simulink library "libbha_io"  (R2015b)
settings: Solver=FixedStepDiscrete  StartTime=0.0  StopTime=Inf  FixedStep=0.004  RelTol=1e-3
PostLoadFcn:
  | , if any(exist('dsrtsu_mdlpostloadfcn', 'file') == [2, 3, 6]), try dsrtsu_mdlpostloadfcn('Execute', bdroot); catch fprintf('Error in PostLoadFcn (dsrtsu_mdlpostloadfcn) for model "%s":\n %s\n', bdroot, lasterr); end, end,
libraries: libbha_io x33, libc_filters_diff x8, libc_bitoperations x8, simulink x7
settings Model: DSRTSU_INTERNAL_RTI_VER=470  DSRTSU_INTERNAL_RTI_TYPE=rti1007  DSRTSU_INTERNAL_RTIFPGA=60  Creator=Falkenhahn  LastModifiedBy=fav
settings DataIOCC: SaveFormat=Array
settings OptimizationCC: BlockReduction=off  OptimizeBlockIOStorage=off  BufferReuse=off  GlobalBufferReuse=off  ExpressionFolding=off  LocalBlockOutputs=off
settings DebuggingCC: UnderspecifiedInitializationDetection=Classic  MergeDetectMultiDrivingBlocksExec=none  SolverPrmCheckMsg=warning
settings HardwareCC: ProdBitPerPointer=32  ProdLargestAtomicFloat=None  ProdEndianess=BigEndian  ProdWordSize=32  ProdHWDeviceType=Generic->Custom  TargetIntDivRoundTo=Zero  TargetEndianess=BigEndian  TargetHWDeviceType=Generic->Custom
settings RTWCC: SystemTargetFile=rti1007.tlc  MakeCommand=make_rti  TemplateMakefile=rti1007.tmf  Description=dSPACE DS1007 Hardware Platform
settings STFCustomTargetCC: ParMdlRefBuildCompliant=on  ConcurrentExecutionCompliant=off  MatFileLogging=on  SystemTargetFile=rti1007.tlc
settings GRTTargetCC: CompOptLevelCompliant=off  ConcurrentExecutionCompliant=off  GeneratePreprocessorConditionals=Disable all  CombineOutputUpdateFcns=off  GRTInterface=on  UseToolchainInfoCompliant=off  ExtModeMexFile=noextcomm
settings ConfigComp: CovModelRefEnable=Off

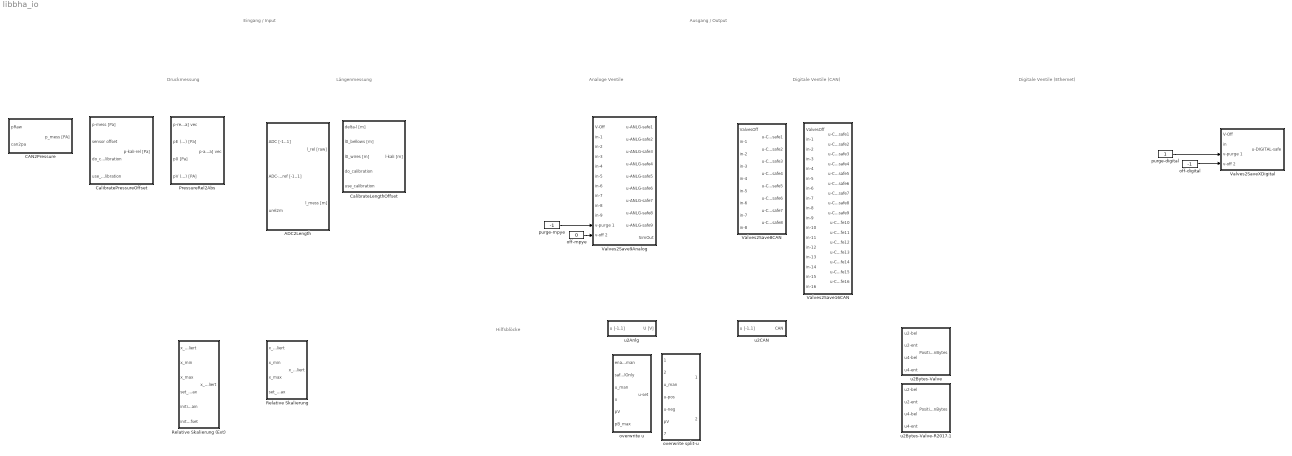
== system libbha_io ==
  note: Druckmessung
  note: Längenmessung
  note: Analoge Ventile
  note: Digitale Ventile (CAN)
  note: Hilfsblöcke
  note: Eingang / Input
  note: Ausgang / Output
  note: Digitale Ventile (Ethernet)
  ADC2Length : Subsystem
  CAN2Pressure : Subsystem
  CalibrateLengthOffset : Subsystem
  CalibratePressureOffset : Subsystem
  PressureRel2Abs : Subsystem
  Relative Skalierung : Subsystem  mask{x_min_init=1e5, x_max_init=2e5}
      mask prompts: x_min_init "x min init"; x_max_init "x max init"
      settings: AttributesFormatString=|
      | Quick-and-dirty Kalibrierung:
      | Passt unskalierte Messgrößen
      | in Zuständen entlüftet (-1) und belüftet (1)
      | auf Minimal- bzw. Maximalwert an
      | 
      | Initialisierung verbesserungswürdig
  Relative Skalierung (Ext) : Subsystem  mask{x_min_init=1e5, x_max_init=2e5}
      mask prompts: x_min_init "x min init"; x_max_init "x max init"
      settings: AttributesFormatString=|
      | Quick-and-dirty Kalibrierung:
      | Passt unskalierte Messgrößen
      | in Zuständen entlüftet (-1) und belüftet (1)
      | auf Minimal- bzw. Maximalwert an
  Valves2Save16CAN : Subsystem
  Valves2Save8CAN : Subsystem
  Valves2Save9Analog : Subsystem
  Valves2SaveXDigital : Subsystem
  off-digital : Constant  Value=-1
  off-mpye : Constant  Value=0
      settings: AttributesFormatString=|
      | mpye: 0
      | mhe: -1 (ambient)
  overwrite split-u : Subsystem
  overwrite u : Subsystem
  purge-digital : Constant
  purge-mpye : Constant  Value=-1
      settings: AttributesFormatString=|
      | mpye -1
      | mhe: 1
  u2Anlg : Subsystem
  u2Bytes-Valve : Subsystem
  u2Bytes-Valve-R2017.1 : Subsystem
  u2CAN : Subsystem
  wires:
  purge-mpye/1 -> Valves2Save9Analog/11(v-purge 1)
  off-mpye/1 -> Valves2Save9Analog/12(v-off 2)
  purge-digital/1 -> Valves2SaveXDigital/3(v-purge 1)
  off-digital/1 -> Valves2SaveXDigital/4(v-off 2)

== system libbha_io/ADC2Length ==
  ADC [-1..1] : Inport
  ADC-U-ref [-1..1] : Inport  Port=2
  urel2m : Inport  Port=3
  Divide : Product  Inputs=*/
  Product : Product  RndMeth=Zero
  Saturation > 0 : Saturate  UpperLimit=inf  LowerLimit=0.001
  l_rel [raw] : Outport
  l_mess [m] : Outport  Port=2
  wires:
  urel2m/1 -> Product/2
  Divide/1 -> Product/1, l_rel [raw]/1
  Product/1 -> l_mess [m]/1
  Saturation > 0/1 -> Divide/2
  ADC [-1..1]/1 -> Divide/1
  ADC-U-ref [-1..1]/1 -> Saturation > 0/1

== system libbha_io/CAN2Pressure ==
  pRaw : Inport
  can2pa : Inport  Port=2
  Data Type Conversion : DataTypeConversion  OutDataTypeStr=double  RndMeth=Nearest
  Product : Product  RndMeth=Zero
  p_mess [PA] : Outport
  wires:
  Product/1 -> p_mess [PA]/1
  can2pa/1 -> Product/2
  Data Type Conversion/1 -> Product/1
  pRaw/1 -> Data Type Conversion/1

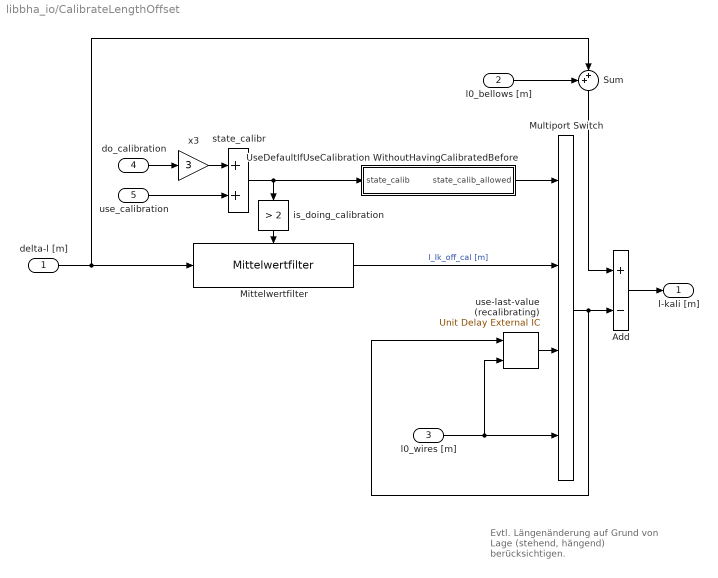
== system libbha_io/CalibrateLengthOffset ==
  note: Evtl. Längenänderung auf Grund von
      | Lage (stehend, hängend) berücksichtigen.
  delta-l [m] : Inport
  l0_bellows [m] : Inport  Port=2
  l0_wires [m] : Inport  Port=3
  do_calibration : Inport  Port=4
  use_calibration : Inport  Port=5
  Add : Sum  Inputs=+-
  Mittelwertfilter : libc_filters_diff/Mittelwertfilter
      settings: AttributesFormatString=Eingangs-Mittelwertbildung wenn aktiviert,\nandernfalls wird Mittelwert gehalten & ausgegeben
  Multiport Switch : MultiPortSwitch  Inputs=2  DataPortForDefault=Additional data port  DiagnosticForDefault=None
  Sum : Sum  Inputs=++|
  UseDefaultIfUseCalibration WithoutHavingCalibratedBefore : Subsystem
  is_doing_calibration : simulink/Logic and Bit Operations/Compare To Constant  relop=>  const=2  OutDataTypeStr=uint8
  state_calibr : Sum
      settings: AttributesFormatString=|
      | 0 = use default
      | 1 = use calibration
      | 2 > do calibration
  use-last-value (recalibrating) : simulink/Additional Math & Discrete/Additional Discrete/Unit Delay External IC  tsamp=-1
  x3 : Gain  Gain=3
  "l-kali [m] " : Outport
  wires:
  use-last-value (recalibrating)/1 -> Multiport Switch/3
  is_doing_calibration/1 -> Mittelwertfilter/Enable
  l0_wires [m]/1 -> use-last-value (recalibrating)/2, Multiport Switch/4
  Multiport Switch/1 -> use-last-value (recalibrating)/1, Add/2
  state_calibr/1 -> UseDefaultIfUseCalibration WithoutHavingCalibratedBefore/1(state_calib), is_doing_calibration/1
  delta-l [m]/1 -> Mittelwertfilter/1, Sum/2
  do_calibration/1 -> x3/1
  x3/1 -> state_calibr/1
  use_calibration/1 -> state_calibr/2
  Add/1 -> "l-kali [m] "/1
  Mittelwertfilter/1 -> Multiport Switch/2  "l_Ik_off_cal [m]"
  Sum/1 -> Add/1
  l0_bellows [m]/1 -> Sum/1
  UseDefaultIfUseCalibration WithoutHavingCalibratedBefore/1(state_calib_allowed) -> Multiport Switch/1

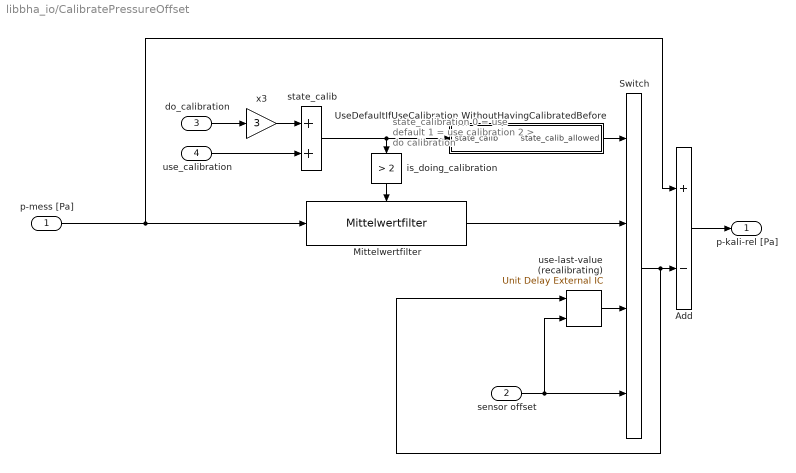
== system libbha_io/CalibratePressureOffset ==
  note: state_calibration
      | 0 = use default
      | 1 = use calibration
      | 2 > do calibration
  p-mess [Pa] : Inport
  sensor offset : Inport  Port=2
  do_calibration : Inport  Port=3
  use_calibration : Inport  Port=4
  Add : Sum  Inputs=+-
  Mittelwertfilter : libc_filters_diff/Mittelwertfilter
      settings: AttributesFormatString=Eingangs-Mittelwertbildung wenn aktiviert,\nandernfalls wird Mittelwert gehalten & ausgegeben
  Switch : MultiPortSwitch  Inputs=2  DataPortForDefault=Additional data port  DiagnosticForDefault=None
  UseDefaultIfUseCalibration WithoutHavingCalibratedBefore : Subsystem
  is_doing_calibration : simulink/Logic and Bit Operations/Compare To Constant  relop=>  const=2  OutDataTypeStr=uint8
  state_calib : Sum
  use-last-value (recalibrating) : simulink/Additional Math & Discrete/Additional Discrete/Unit Delay External IC  tsamp=-1
  x3 : Gain  Gain=3
  p-kali-rel [Pa] : Outport
  wires:
  use_calibration/1 -> state_calib/2
  x3/1 -> state_calib/1
  state_calib/1 -> UseDefaultIfUseCalibration WithoutHavingCalibratedBefore/1(state_calib), is_doing_calibration/1
  Switch/1 -> use-last-value (recalibrating)/1, Add/2
  sensor offset/1 -> use-last-value (recalibrating)/2, Switch/4
  Mittelwertfilter/1 -> Switch/2
  is_doing_calibration/1 -> Mittelwertfilter/Enable
  use-last-value (recalibrating)/1 -> Switch/3
  UseDefaultIfUseCalibration WithoutHavingCalibratedBefore/1(state_calib_allowed) -> Switch/1
  Add/1 -> p-kali-rel [Pa]/1
  p-mess [Pa]/1 -> Mittelwertfilter/1, Add/1
  do_calibration/1 -> x3/1

== system libbha_io/PressureRel2Abs ==
  p-rel [Pa] vec : Inport
  pE (min) [Pa] : Inport  Port=2
  p0 [Pa] : Inport  Port=3
  pV (max) [PA] : Inport  Port=4
  Saturation Dynamic : simulink/Discontinuities/Saturation Dynamic  OutMin=[]  OutMax=[]  OutDataTypeStr=Inherit: Same as second input  OutDataType=fixdt(1, 16)  OutScaling=2^-10  DoSatur=off
  Sum : Sum  Inputs=|++
  do not allow pressures close to zero : Saturate  UpperLimit=inf  LowerLimit=0.11e5
  p-abs [Pa] vec : Outport
  wires:
  do not allow pressures close to zero/1 -> p-abs [Pa] vec/1
  Saturation Dynamic/1 -> do not allow pressures close to zero/1
  p0 [Pa]/1 -> Sum/2
  Sum/1 -> Saturation Dynamic/2
  pV (max) [PA]/1 -> Saturation Dynamic/1
  p-rel [Pa] vec/1 -> Sum/1  "l_meas_11"
  pE (min) [Pa]/1 -> Saturation Dynamic/3

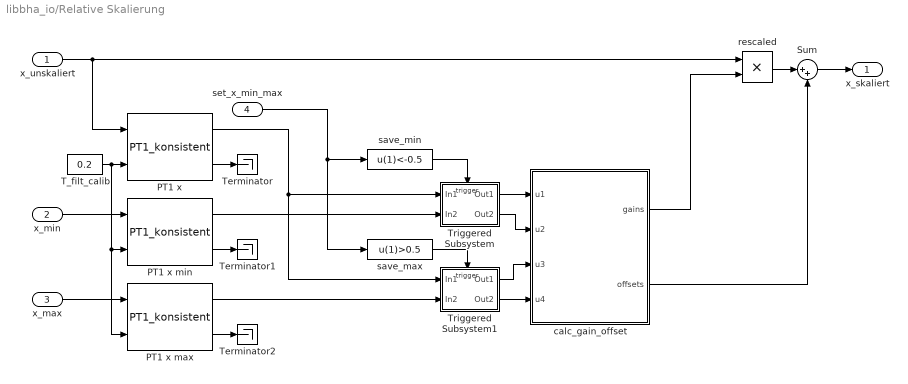
== system libbha_io/Relative Skalierung ==
  x_unskaliert : Inport
  x_min : Inport  Port=2
  x_max : Inport  Port=3
  set_x_min_max : Inport  Port=4
  PT1 x : libc_filters_diff/PT1_konsistent
  PT1 x max : libc_filters_diff/PT1_konsistent
  PT1 x min : libc_filters_diff/PT1_konsistent
  Sum : Sum  Inputs=|++
  T_filt_calib : Constant  Value=0.2
  Terminator : Terminator
  Terminator1 : Terminator
  Terminator2 : Terminator
  Triggered Subsystem : Subsystem  TreatAsAtomicUnit=on
  Triggered Subsystem1 : Subsystem  TreatAsAtomicUnit=on
  calc_gain_offset : MATLAB Function  TreatAsAtomicUnit=on
  rescaled : Product  Inputs=**  RndMeth=Zero
  save_max : Fcn  Expr=u(1)>0.5
  save_min : Fcn  Expr=u(1)<-0.5
  x_skaliert : Outport
  wires:
  PT1 x/1 -> Triggered Subsystem/1(In1), Triggered Subsystem1/1(In1)
  x_min/1 -> PT1 x min/1
  save_max/1 -> Triggered Subsystem1/Trigger
  x_unskaliert/1 -> PT1 x/1, rescaled/1
  set_x_min_max/1 -> save_max/1, save_min/1
  rescaled/1 -> Sum/1
  Sum/1 -> x_skaliert/1
  calc_gain_offset/1(gains) -> rescaled/2
  calc_gain_offset/2(offsets) -> Sum/2
  PT1 x min/1 -> Triggered Subsystem/2(In2)
  PT1 x max/1 -> Triggered Subsystem1/2(In2)
  save_min/1 -> Triggered Subsystem/Trigger
  x_max/1 -> PT1 x max/1
  T_filt_calib/1 -> PT1 x min/2, PT1 x max/2, PT1 x/2
  PT1 x/2 -> Terminator/1
  PT1 x min/2 -> Terminator1/1
  PT1 x max/2 -> Terminator2/1
  Triggered Subsystem/1(Out1) -> calc_gain_offset/1(u1)
  Triggered Subsystem/2(Out2) -> calc_gain_offset/2(u2)
  Triggered Subsystem1/2(Out2) -> calc_gain_offset/4(u4)
  Triggered Subsystem1/1(Out1) -> calc_gain_offset/3(u3)

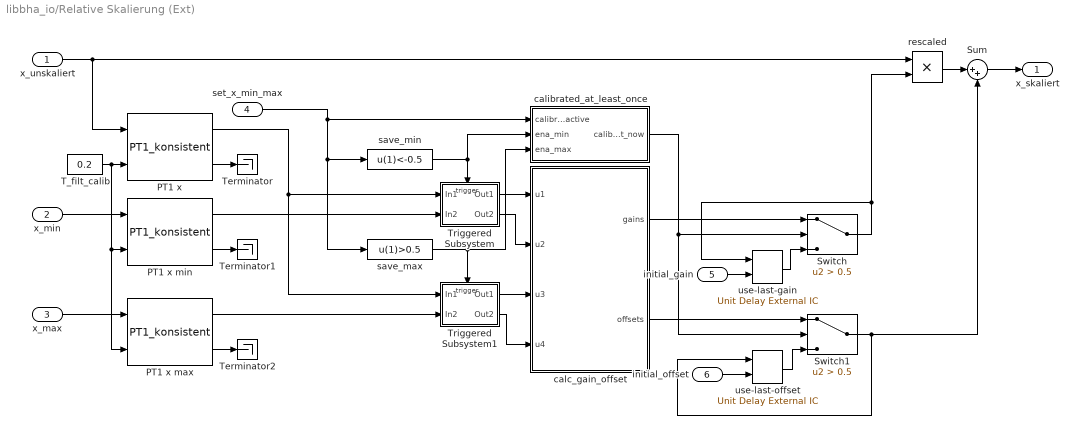
== system libbha_io/Relative Skalierung (Ext) ==
  x_unskaliert : Inport
  x_min : Inport  Port=2
  x_max : Inport  Port=3
  set_x_min_max : Inport  Port=4
  initial_gain : Inport  Port=5
  initial_offset : Inport  Port=6
  PT1 x : libc_filters_diff/PT1_konsistent
  PT1 x max : libc_filters_diff/PT1_konsistent
  PT1 x min : libc_filters_diff/PT1_konsistent
  Sum : Sum  Inputs=|++
  Switch : Switch  Criteria=u2 > Threshold  Threshold=0.5
  Switch1 : Switch  Criteria=u2 > Threshold  Threshold=0.5
  T_filt_calib : Constant  Value=0.2
  Terminator : Terminator
  Terminator1 : Terminator
  Terminator2 : Terminator
  Triggered Subsystem : Subsystem  TreatAsAtomicUnit=on
  Triggered Subsystem1 : Subsystem  TreatAsAtomicUnit=on
  calc_gain_offset : MATLAB Function  TreatAsAtomicUnit=on
  calibrated_at_least_once : Subsystem
  rescaled : Product  Inputs=**  RndMeth=Zero
  save_max : Fcn  Expr=u(1)>0.5
  save_min : Fcn  Expr=u(1)<-0.5
  use-last-gain : simulink/Additional Math & Discrete/Additional Discrete/Unit Delay External IC  tsamp=-1
  use-last-offset : simulink/Additional Math & Discrete/Additional Discrete/Unit Delay External IC  tsamp=-1
  x_skaliert : Outport
  wires:
  Triggered Subsystem1/1(Out1) -> calc_gain_offset/3(u3)
  Triggered Subsystem1/2(Out2) -> calc_gain_offset/4(u4)
  Triggered Subsystem/2(Out2) -> calc_gain_offset/2(u2)
  Triggered Subsystem/1(Out1) -> calc_gain_offset/1(u1)
  PT1 x max/2 -> Terminator2/1
  PT1 x min/2 -> Terminator1/1
  PT1 x/2 -> Terminator/1
  T_filt_calib/1 -> PT1 x/2, PT1 x max/2, PT1 x min/2
  x_max/1 -> PT1 x max/1
  save_min/1 -> calibrated_at_least_once/2(ena_min), Triggered Subsystem/Trigger
  PT1 x max/1 -> Triggered Subsystem1/2(In2)
  PT1 x min/1 -> Triggered Subsystem/2(In2)
  Switch1/1 -> Sum/2, use-last-offset/1
  Switch/1 -> rescaled/2, use-last-gain/1
  Sum/1 -> x_skaliert/1
  rescaled/1 -> Sum/1
  set_x_min_max/1 -> save_min/1, save_max/1, calibrated_at_least_once/1(calibration_active)
  x_unskaliert/1 -> rescaled/1, PT1 x/1
  save_max/1 -> calibrated_at_least_once/3(ena_max), Triggered Subsystem1/Trigger
  x_min/1 -> PT1 x min/1
  PT1 x/1 -> Triggered Subsystem1/1(In1), Triggered Subsystem/1(In1)
  initial_gain/1 -> use-last-gain/2
  calc_gain_offset/1(gains) -> Switch/1
  calibrated_at_least_once/1(calib_once_not_now) -> Switch1/2, Switch/2
  use-last-gain/1 -> Switch/3
  calc_gain_offset/2(offsets) -> Switch1/1
  initial_offset/1 -> use-last-offset/2
  use-last-offset/1 -> Switch1/3

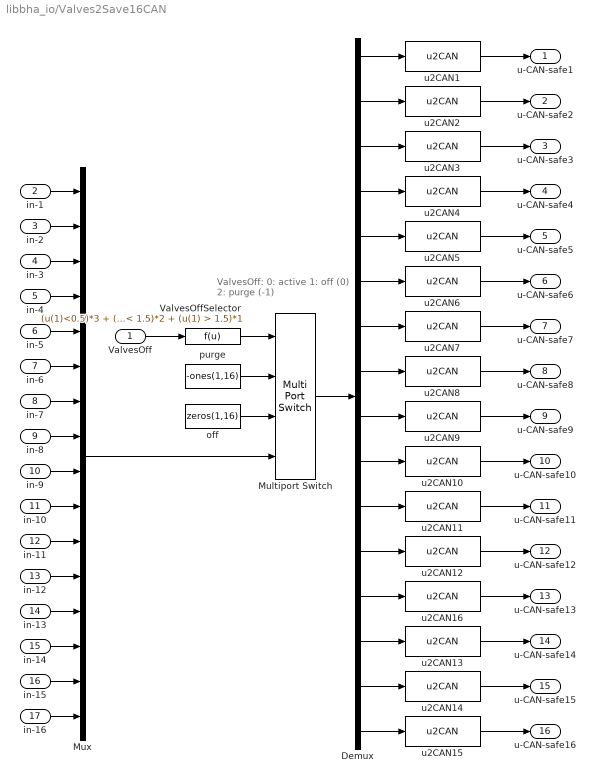
== system libbha_io/Valves2Save16CAN ==
  note: ValvesOff:
      | 0: active
      | 1: off (0)
      | 2: purge (-1)
  ValvesOff : Inport
  in-1 : Inport  Port=2
  in-2 : Inport  Port=3
  in-3 : Inport  Port=4
  in-4 : Inport  Port=5
  in-5 : Inport  Port=6
  in-6 : Inport  Port=7
  in-7 : Inport  Port=8
  in-8 : Inport  Port=9
  in-9 : Inport  Port=10
  in-10 : Inport  Port=11
  in-11 : Inport  Port=12
  in-12 : Inport  Port=13
  in-13 : Inport  Port=14
  in-14 : Inport  Port=15
  in-15 : Inport  Port=16
  in-16 : Inport  Port=17
  Demux : Demux  Outputs=16
  Multiport Switch : MultiPortSwitch
  Mux : Mux  Inputs=16
  ValvesOffSelector : Fcn  Expr=(u(1)<0.5)*3 + (u(1) >0.5)*(u(1) < 1.5)*2 + (u(1) > 1.5)*1
  off : Constant  Value=zeros(1,16)
  purge : Constant  Value=-ones(1,16)
  u2CAN{1..16} (16 alike) : libbha_io/u2CAN
  u-CAN-safe1 : Outport
  u-CAN-safe2 : Outport  Port=2
  u-CAN-safe3 : Outport  Port=3
  u-CAN-safe4 : Outport  Port=4
  u-CAN-safe5 : Outport  Port=5
  u-CAN-safe6 : Outport  Port=6
  u-CAN-safe7 : Outport  Port=7
  u-CAN-safe8 : Outport  Port=8
  u-CAN-safe9 : Outport  Port=9
  u-CAN-safe10 : Outport  Port=10
  u-CAN-safe11 : Outport  Port=11
  u-CAN-safe12 : Outport  Port=12
  u-CAN-safe13 : Outport  Port=13
  u-CAN-safe14 : Outport  Port=14
  u-CAN-safe15 : Outport  Port=15
  u-CAN-safe16 : Outport  Port=16
  wires:
  u2CAN8/1 -> u-CAN-safe8/1
  u2CAN7/1 -> u-CAN-safe7/1
  u2CAN6/1 -> u-CAN-safe6/1
  u2CAN5/1 -> u-CAN-safe5/1
  u2CAN4/1 -> u-CAN-safe4/1
  u2CAN3/1 -> u-CAN-safe3/1
  u2CAN2/1 -> u-CAN-safe2/1
  u2CAN1/1 -> u-CAN-safe1/1
  Demux/8 -> u2CAN8/1
  Demux/7 -> u2CAN7/1
  Demux/6 -> u2CAN6/1
  Demux/5 -> u2CAN5/1
  Demux/4 -> u2CAN4/1
  Demux/3 -> u2CAN3/1
  Demux/2 -> u2CAN2/1
  Demux/1 -> u2CAN1/1
  in-8/1 -> Mux/8
  in-7/1 -> Mux/7
  in-6/1 -> Mux/6
  in-5/1 -> Mux/5
  in-4/1 -> Mux/4
  in-3/1 -> Mux/3
  in-2/1 -> Mux/2
  in-1/1 -> Mux/1
  ValvesOff/1 -> ValvesOffSelector/1
  Mux/1 -> Multiport Switch/4
  Multiport Switch/1 -> Demux/1
  off/1 -> Multiport Switch/3
  purge/1 -> Multiport Switch/2
  ValvesOffSelector/1 -> Multiport Switch/1
  in-9/1 -> Mux/9
  in-10/1 -> Mux/10
  in-11/1 -> Mux/11
  in-12/1 -> Mux/12
  in-13/1 -> Mux/13
  in-14/1 -> Mux/14
  in-15/1 -> Mux/15
  in-16/1 -> Mux/16
  u2CAN9/1 -> u-CAN-safe9/1
  Demux/9 -> u2CAN9/1
  u2CAN10/1 -> u-CAN-safe10/1
  u2CAN11/1 -> u-CAN-safe11/1
  u2CAN12/1 -> u-CAN-safe12/1
  u2CAN16/1 -> u-CAN-safe13/1
  u2CAN13/1 -> u-CAN-safe14/1
  u2CAN14/1 -> u-CAN-safe15/1
  u2CAN15/1 -> u-CAN-safe16/1
  Demux/10 -> u2CAN10/1
  Demux/11 -> u2CAN11/1
  Demux/12 -> u2CAN12/1
  Demux/13 -> u2CAN16/1
  Demux/14 -> u2CAN13/1
  Demux/15 -> u2CAN14/1
  Demux/16 -> u2CAN15/1

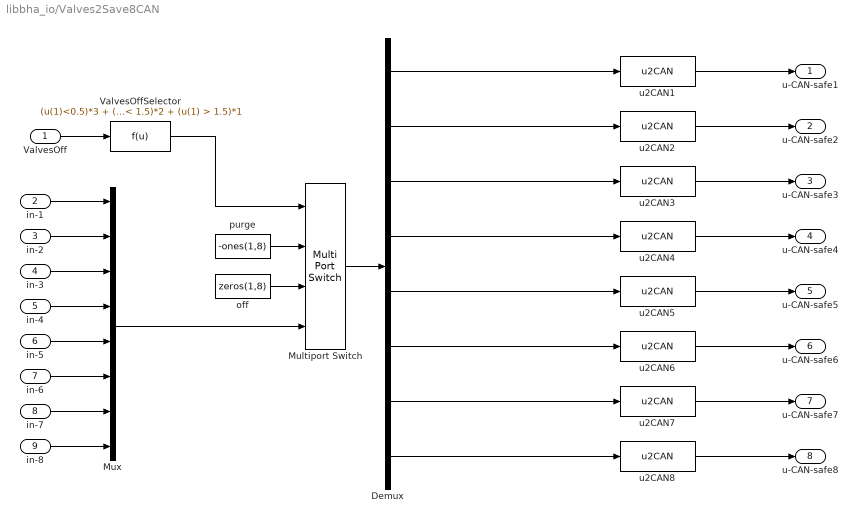
== system libbha_io/Valves2Save8CAN ==
  ValvesOff : Inport
  in-1 : Inport  Port=2
  in-2 : Inport  Port=3
  in-3 : Inport  Port=4
  in-4 : Inport  Port=5
  in-5 : Inport  Port=6
  in-6 : Inport  Port=7
  in-7 : Inport  Port=8
  in-8 : Inport  Port=9
  Demux : Demux  Outputs=8
  Multiport Switch : MultiPortSwitch
  Mux : Mux  Inputs=8
  ValvesOffSelector : Fcn  Expr=(u(1)<0.5)*3 + (u(1) >0.5)*(u(1) < 1.5)*2 + (u(1) > 1.5)*1
  off : Constant  Value=zeros(1,8)
  purge : Constant  Value=-ones(1,8)
  u2CAN{1..8} (8 alike) : libbha_io/u2CAN
  u-CAN-safe1 : Outport
  u-CAN-safe2 : Outport  Port=2
  u-CAN-safe3 : Outport  Port=3
  u-CAN-safe4 : Outport  Port=4
  u-CAN-safe5 : Outport  Port=5
  u-CAN-safe6 : Outport  Port=6
  u-CAN-safe7 : Outport  Port=7
  u-CAN-safe8 : Outport  Port=8
  wires:
  ValvesOffSelector/1 -> Multiport Switch/1
  purge/1 -> Multiport Switch/2
  off/1 -> Multiport Switch/3
  Multiport Switch/1 -> Demux/1
  Mux/1 -> Multiport Switch/4
  ValvesOff/1 -> ValvesOffSelector/1
  in-1/1 -> Mux/1
  in-2/1 -> Mux/2
  in-3/1 -> Mux/3
  in-4/1 -> Mux/4
  in-5/1 -> Mux/5
  in-6/1 -> Mux/6
  in-7/1 -> Mux/7
  in-8/1 -> Mux/8
  Demux/1 -> u2CAN1/1
  Demux/2 -> u2CAN2/1
  Demux/3 -> u2CAN3/1
  Demux/4 -> u2CAN4/1
  Demux/5 -> u2CAN5/1
  Demux/6 -> u2CAN6/1
  Demux/7 -> u2CAN7/1
  Demux/8 -> u2CAN8/1
  u2CAN1/1 -> u-CAN-safe1/1
  u2CAN2/1 -> u-CAN-safe2/1
  u2CAN3/1 -> u-CAN-safe3/1
  u2CAN4/1 -> u-CAN-safe4/1
  u2CAN5/1 -> u-CAN-safe5/1
  u2CAN6/1 -> u-CAN-safe6/1
  u2CAN7/1 -> u-CAN-safe7/1
  u2CAN8/1 -> u-CAN-safe8/1

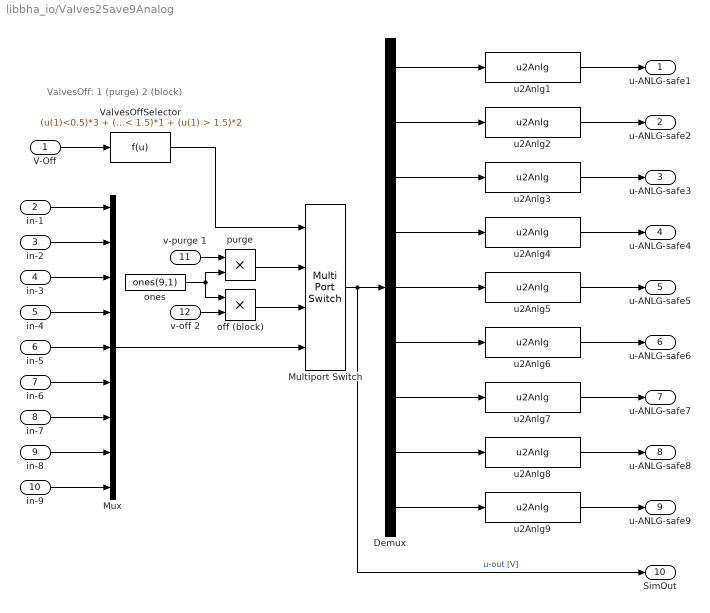
== system libbha_io/Valves2Save9Analog ==
  note: ValvesOff:
      | 1 (purge)
      | 2 (block)
  V-Off : Inport
  in-1 : Inport  Port=2
  in-2 : Inport  Port=3
  in-3 : Inport  Port=4
  in-4 : Inport  Port=5
  in-5 : Inport  Port=6
  in-6 : Inport  Port=7
  in-7 : Inport  Port=8
  in-8 : Inport  Port=9
  in-9 : Inport  Port=10
  v-purge 1 : Inport  Port=11
  v-off 2 : Inport  Port=12
  Demux : Demux  Outputs=9
  Multiport Switch : MultiPortSwitch
  Mux : Mux  Inputs=9
  ValvesOffSelector : Fcn  Expr=(u(1)<0.5)*3 + (u(1) >0.5)*(u(1) < 1.5)*1 + (u(1) > 1.5)*2
  off (block) : Product  RndMeth=Zero
  ones : Constant  Value=ones(9,1)
  purge : Product  RndMeth=Zero
  u2Anlg{1..9} (9 alike) : libbha_io/u2Anlg
  u-ANLG-safe1 : Outport
  u-ANLG-safe2 : Outport  Port=2
  u-ANLG-safe3 : Outport  Port=3
  u-ANLG-safe4 : Outport  Port=4
  u-ANLG-safe5 : Outport  Port=5
  u-ANLG-safe6 : Outport  Port=6
  u-ANLG-safe7 : Outport  Port=7
  u-ANLG-safe8 : Outport  Port=8
  u-ANLG-safe9 : Outport  Port=9
  SimOut : Outport  Port=10
  wires:
  v-off 2/1 -> off (block)/2
  v-purge 1/1 -> purge/1
  ones/1 -> purge/2, off (block)/1
  u2Anlg1/1 -> u-ANLG-safe1/1
  Demux/8 -> u2Anlg8/1
  Demux/7 -> u2Anlg7/1
  Demux/6 -> u2Anlg6/1
  Demux/5 -> u2Anlg5/1
  Demux/4 -> u2Anlg4/1
  Demux/3 -> u2Anlg3/1
  Demux/2 -> u2Anlg2/1
  Demux/1 -> u2Anlg1/1
  in-8/1 -> Mux/8
  in-7/1 -> Mux/7
  in-6/1 -> Mux/6
  in-5/1 -> Mux/5
  in-4/1 -> Mux/4
  in-3/1 -> Mux/3
  in-2/1 -> Mux/2
  in-1/1 -> Mux/1
  V-Off/1 -> ValvesOffSelector/1
  Mux/1 -> Multiport Switch/4
  Multiport Switch/1 -> SimOut/1, Demux/1  "u-out [V]"
  off (block)/1 -> Multiport Switch/3
  purge/1 -> Multiport Switch/2
  ValvesOffSelector/1 -> Multiport Switch/1
  in-9/1 -> Mux/9
  Demux/9 -> u2Anlg9/1
  u2Anlg2/1 -> u-ANLG-safe2/1
  u2Anlg3/1 -> u-ANLG-safe3/1
  u2Anlg4/1 -> u-ANLG-safe4/1
  u2Anlg5/1 -> u-ANLG-safe5/1
  u2Anlg6/1 -> u-ANLG-safe6/1
  u2Anlg7/1 -> u-ANLG-safe7/1
  u2Anlg8/1 -> u-ANLG-safe8/1
  u2Anlg9/1 -> u-ANLG-safe9/1

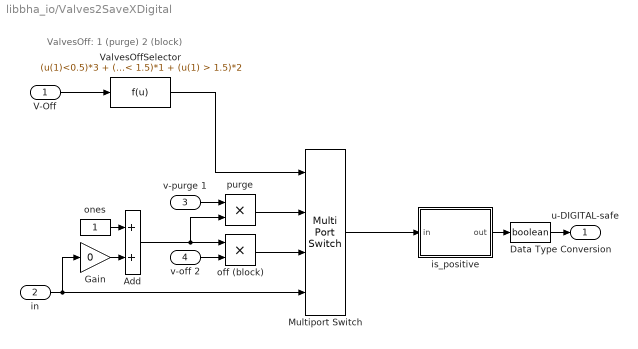
== system libbha_io/Valves2SaveXDigital ==
  note: ValvesOff:
      | 1 (purge)
      | 2 (block)
  V-Off : Inport
  in : Inport  Port=2
  v-purge 1 : Inport  Port=3
  v-off 2 : Inport  Port=4
  Add : Sum
  Data Type Conversion : DataTypeConversion  OutDataTypeStr=boolean
  Gain : Gain  Gain=0
  Multiport Switch : MultiPortSwitch
  ValvesOffSelector : Fcn  Expr=(u(1)<0.5)*3 + (u(1) >0.5)*(u(1) < 1.5)*1 + (u(1) > 1.5)*2
  is_positive : MATLAB Function  TreatAsAtomicUnit=on
      settings: AttributesFormatString=|
      | Ausgang 1: Vakuum
      | Ausgang 0: Umgebung
  off (block) : Product  RndMeth=Zero
  ones : Constant
  purge : Product  RndMeth=Zero
  u-DIGITAL-safe : Outport
  wires:
  ValvesOffSelector/1 -> Multiport Switch/1
  purge/1 -> Multiport Switch/2
  off (block)/1 -> Multiport Switch/3
  Multiport Switch/1 -> is_positive/1(in)
  in/1 -> Gain/1, Multiport Switch/4
  V-Off/1 -> ValvesOffSelector/1
  v-purge 1/1 -> purge/1
  v-off 2/1 -> off (block)/2
  Add/1 -> purge/2, off (block)/1
  Gain/1 -> Add/2
  ones/1 -> Add/1
  is_positive/1(out) -> Data Type Conversion/1
  Data Type Conversion/1 -> u-DIGITAL-safe/1

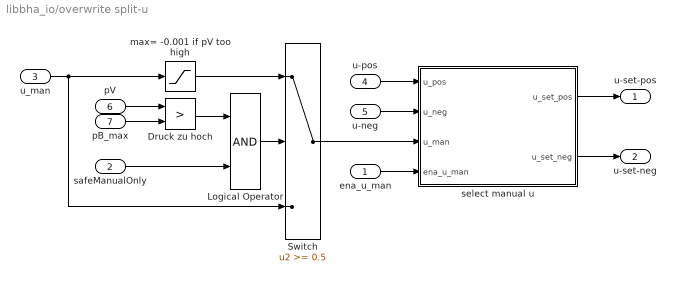
== system libbha_io/overwrite split-u ==
  ena_u_man : Inport
  safeManualOnly : Inport  Port=2
  u_man : Inport  Port=3
  u-pos : Inport  Port=4
  u-neg : Inport  Port=5
  pV : Inport  Port=6
  pB_max : Inport  Port=7
  Druck zu hoch : RelationalOperator  Operator=>  OutDataTypeStr=boolean
  Logical Operator : Logic  AllPortsSameDT=off  OutDataTypeStr=boolean
  Switch : Switch  Threshold=0.5
  max= -0.001 if pV too high : Saturate  UpperLimit=-0.001  LowerLimit=-inf
  select manual u : MATLAB Function  TreatAsAtomicUnit=on
  u-set-pos : Outport
      settings: AttributesFormatString=dimension: -1
  u-set-neg : Outport  Port=2
      settings: AttributesFormatString=dimension: -1
  wires:
  pV/1 -> Druck zu hoch/1
  pB_max/1 -> Druck zu hoch/2
  Logical Operator/1 -> Switch/2
  u_man/1 -> Switch/3, max= -0.001 if pV too high/1
  max= -0.001 if pV too high/1 -> Switch/1
  Switch/1 -> select manual u/3(u_man)
  u-pos/1 -> select manual u/1(u_pos)
  ena_u_man/1 -> select manual u/4(ena_u_man)
  Druck zu hoch/1 -> Logical Operator/1
  safeManualOnly/1 -> Logical Operator/2
  u-neg/1 -> select manual u/2(u_neg)
  select manual u/1(u_set_pos) -> u-set-pos/1
  select manual u/2(u_set_neg) -> u-set-neg/1

== system libbha_io/overwrite u ==
  ena_u_man : Inport
  safeManualOnly : Inport  Port=2
  u_man : Inport  Port=3
  u : Inport  Port=4
  pV : Inport  Port=5
  pB_max : Inport  Port=6
  Druck zu hoch : RelationalOperator  Operator=>  OutDataTypeStr=boolean
  Logical Operator : Logic  AllPortsSameDT=off  OutDataTypeStr=boolean
  Switch : Switch  Threshold=0.5
  max= -0.001 if pV too high : Saturate  UpperLimit=-0.001  LowerLimit=-inf
  select manual u : MATLAB Function  TreatAsAtomicUnit=on
  u-set : Outport  PortDimensions=3
      settings: AttributesFormatString=dimension: 3
  wires:
  safeManualOnly/1 -> Logical Operator/2
  Druck zu hoch/1 -> Logical Operator/1
  select manual u/1(u_set) -> u-set/1
  ena_u_man/1 -> select manual u/3(ena_u_man)
  u/1 -> select manual u/1(u)
  Switch/1 -> select manual u/2(u_man)
  max= -0.001 if pV too high/1 -> Switch/1
  u_man/1 -> max= -0.001 if pV too high/1, Switch/3
  Logical Operator/1 -> Switch/2
  pB_max/1 -> Druck zu hoch/2
  pV/1 -> Druck zu hoch/1

== system libbha_io/u2Anlg ==
  u [-1,1] : Inport
  Convert : Fcn  Expr=(u(1)*5+5)
  Override Switch : MultiPortSwitch  DataPortOrder=Zero-based contiguous  Inputs=2
  Saturation [-1,1] : Saturate  UpperLimit=1  LowerLimit=-1
  override : Constant  Value=0
  override_value : Constant  Value=0.0
  U [V] : Outport
  wires:
  override/1 -> Override Switch/1
  override_value/1 -> Override Switch/3
  u [-1,1]/1 -> Override Switch/2
  Override Switch/1 -> Saturation [-1,1]/1
  Convert/1 -> U [V]/1
  Saturation [-1,1]/1 -> Convert/1

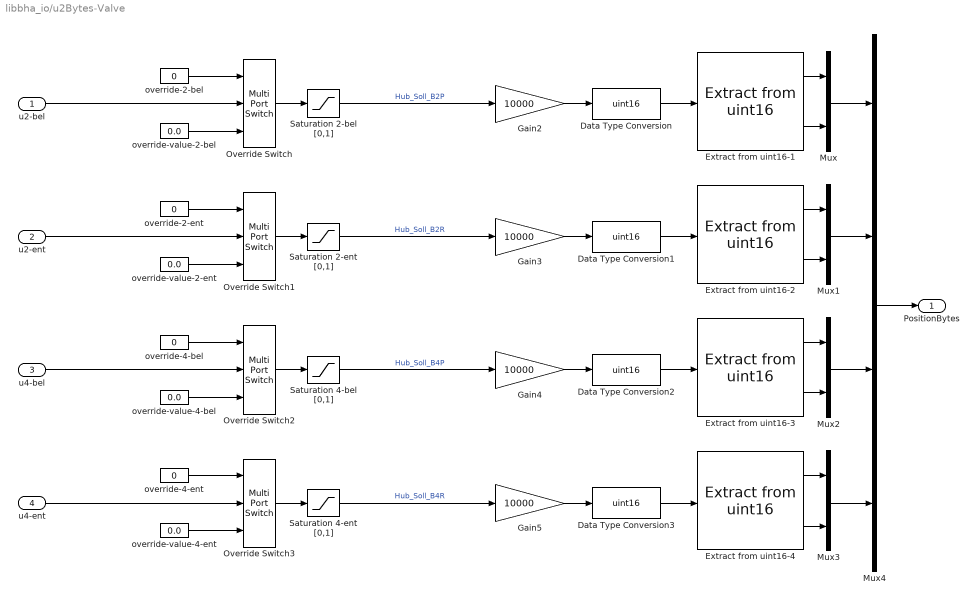
== system libbha_io/u2Bytes-Valve ==
  u2-bel : Inport
      settings: AttributesFormatString=[0,1]
  u2-ent : Inport  Port=2
      settings: AttributesFormatString=[0,1]
  u4-bel : Inport  Port=3
      settings: AttributesFormatString=[0,1]
  u4-ent : Inport  Port=4
      settings: AttributesFormatString=[0,1]
  Data Type Conversion{,1..3} (4 alike) : DataTypeConversion  OutDataTypeStr=uint16
  Extract from uint16-{1..4} (4 alike) : libc_bitoperations/Extract from uint16
  Gain{2..5} (4 alike) : Gain  Gain=10000
  Mux{,1..3} (4 alike) : Mux  Inputs=2
  Mux4 : Mux
  Override Switch{,1..3} (4 alike) : MultiPortSwitch  DataPortOrder=Zero-based contiguous  Inputs=2
  Saturation 2-bel [0,1] : Saturate  UpperLimit=1  LowerLimit=0
  Saturation 2-ent [0,1] : Saturate  UpperLimit=1  LowerLimit=0
  Saturation 4-bel [0,1] : Saturate  UpperLimit=1  LowerLimit=0
  Saturation 4-ent [0,1] : Saturate  UpperLimit=1  LowerLimit=0
  override-2-bel : Constant  Value=0
  override-2-ent : Constant  Value=0
  override-4-bel : Constant  Value=0
  override-4-ent : Constant  Value=0
  override-value-2-bel : Constant  Value=0.0
  override-value-2-ent : Constant  Value=0.0
  override-value-4-bel : Constant  Value=0.0
  override-value-4-ent : Constant  Value=0.0
  PositionBytes : Outport
  wires:
  u4-ent/1 -> Override Switch3/2
  u2-ent/1 -> Override Switch1/2
  Saturation 2-bel [0,1]/1 -> Gain2/1  "Hub_Soll_B2P"
  Mux4/1 -> PositionBytes/1
  Override Switch/1 -> Saturation 2-bel [0,1]/1
  u2-bel/1 -> Override Switch/2
  override-value-2-bel/1 -> Override Switch/3
  override-2-bel/1 -> Override Switch/1
  override-value-2-ent/1 -> Override Switch1/3
  override-2-ent/1 -> Override Switch1/1
  Override Switch1/1 -> Saturation 2-ent [0,1]/1
  Saturation 4-bel [0,1]/1 -> Gain4/1  "Hub_Soll_B4P"
  Override Switch2/1 -> Saturation 4-bel [0,1]/1
  u4-bel/1 -> Override Switch2/2
  override-value-4-bel/1 -> Override Switch2/3
  override-4-bel/1 -> Override Switch2/1
  override-value-4-ent/1 -> Override Switch3/3
  override-4-ent/1 -> Override Switch3/1
  Override Switch3/1 -> Saturation 4-ent [0,1]/1
  Gain2/1 -> Data Type Conversion/1
  Data Type Conversion/1 -> Extract from uint16-1/1
  Extract from uint16-1/2 -> Mux/2
  Extract from uint16-1/1 -> Mux/1
  Saturation 2-ent [0,1]/1 -> Gain3/1  "Hub_Soll_B2R"
  Gain3/1 -> Data Type Conversion1/1
  Data Type Conversion1/1 -> Extract from uint16-2/1
  Extract from uint16-2/2 -> Mux1/2
  Extract from uint16-2/1 -> Mux1/1
  Gain4/1 -> Data Type Conversion2/1
  Data Type Conversion2/1 -> Extract from uint16-3/1
  Extract from uint16-3/2 -> Mux2/2
  Extract from uint16-3/1 -> Mux2/1
  Gain5/1 -> Data Type Conversion3/1
  Data Type Conversion3/1 -> Extract from uint16-4/1
  Extract from uint16-4/2 -> Mux3/2
  Extract from uint16-4/1 -> Mux3/1
  Saturation 4-ent [0,1]/1 -> Gain5/1  "Hub_Soll_B4R"
  Mux2/1 -> Mux4/3
  Mux1/1 -> Mux4/2
  Mux3/1 -> Mux4/4
  Mux/1 -> Mux4/1

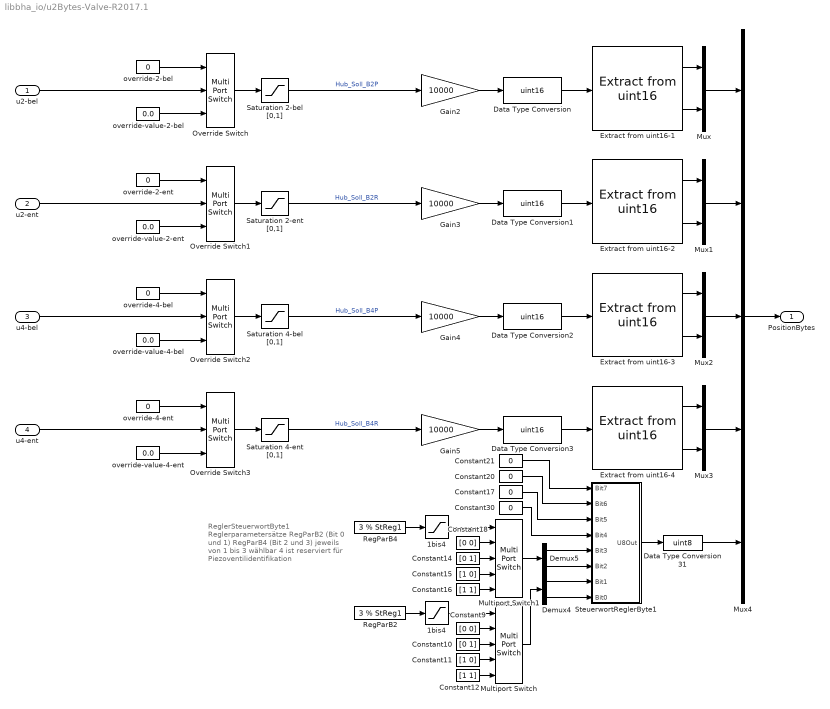
== system libbha_io/u2Bytes-Valve-R2017.1 ==
  note: ReglerSteuerwortByte1
      | Reglerparametersätze
      |  RegParB2 (Bit 0 und 1)
      |  RegParB4 (Bit 2 und 3)
      | jeweils von 1 bis 3 wählbar
      | 4 ist reserviert für Piezoventilidentifikation
  u2-bel : Inport
      settings: AttributesFormatString=[0,1]
  u2-ent : Inport  Port=2
      settings: AttributesFormatString=[0,1]
  u4-bel : Inport  Port=3
      settings: AttributesFormatString=[0,1]
  u4-ent : Inport  Port=4
      settings: AttributesFormatString=[0,1]
  1bis4 : Saturate  UpperLimit=4  LowerLimit=1
  "1bis4 " : Saturate  UpperLimit=4  LowerLimit=1
  Constant10 : Constant  Value=[0 1]
  Constant11 : Constant  Value=[1 0]
  Constant12 : Constant  Value=[1 1]
  Constant14 : Constant  Value=[0 1]
  Constant15 : Constant  Value=[1 0]
  Constant16 : Constant  Value=[1 1]
  Constant{17,20..21,30} (4 alike) : Constant  Value=0
  Constant18 : Constant  Value=[0 0]
  Constant9 : Constant  Value=[0 0]
  Data Type Conversion{,1..3} (4 alike) : DataTypeConversion  OutDataTypeStr=uint16
  Data Type Conversion31 : DataTypeConversion  OutDataTypeStr=uint8  RndMeth=Nearest
  Demux4 : Demux  Outputs=2
  Demux5 : Demux  Outputs=2
  Extract from uint16-{1..4} (4 alike) : libc_bitoperations/Extract from uint16
  Gain{2..5} (4 alike) : Gain  Gain=10000
  Multiport Switch : MultiPortSwitch  Inputs=4
  Multiport Switch1 : MultiPortSwitch  Inputs=4
  Mux{,1..3} (4 alike) : Mux  Inputs=2
  Mux4 : Mux  Inputs=5
  Override Switch{,1..3} (4 alike) : MultiPortSwitch  DataPortOrder=Zero-based contiguous  Inputs=2
  RegParB2 : Constant  Value=3 % StReg1
  RegParB4 : Constant  Value=3 % StReg1
  Saturation 2-bel [0,1] : Saturate  UpperLimit=1  LowerLimit=0
  Saturation 2-ent [0,1] : Saturate  UpperLimit=1  LowerLimit=0
  Saturation 4-bel [0,1] : Saturate  UpperLimit=1  LowerLimit=0
  Saturation 4-ent [0,1] : Saturate  UpperLimit=1  LowerLimit=0
  SteuerwortReglerByte1 : Subsystem
  override-2-bel : Constant  Value=0
  override-2-ent : Constant  Value=0
  override-4-bel : Constant  Value=0
  override-4-ent : Constant  Value=0
  override-value-2-bel : Constant  Value=0.0
  override-value-2-ent : Constant  Value=0.0
  override-value-4-bel : Constant  Value=0.0
  override-value-4-ent : Constant  Value=0.0
  PositionBytes : Outport
  wires:
  Mux/1 -> Mux4/1
  Mux3/1 -> Mux4/4
  Mux1/1 -> Mux4/2
  Mux2/1 -> Mux4/3
  Saturation 4-ent [0,1]/1 -> Gain5/1  "Hub_Soll_B4R"
  Extract from uint16-4/1 -> Mux3/1
  Extract from uint16-4/2 -> Mux3/2
  Data Type Conversion3/1 -> Extract from uint16-4/1
  Gain5/1 -> Data Type Conversion3/1
  Extract from uint16-3/1 -> Mux2/1
  Extract from uint16-3/2 -> Mux2/2
  Data Type Conversion2/1 -> Extract from uint16-3/1
  Gain4/1 -> Data Type Conversion2/1
  Extract from uint16-2/1 -> Mux1/1
  Extract from uint16-2/2 -> Mux1/2
  Data Type Conversion1/1 -> Extract from uint16-2/1
  Gain3/1 -> Data Type Conversion1/1
  Saturation 2-ent [0,1]/1 -> Gain3/1  "Hub_Soll_B2R"
  Extract from uint16-1/1 -> Mux/1
  Extract from uint16-1/2 -> Mux/2
  Data Type Conversion/1 -> Extract from uint16-1/1
  Gain2/1 -> Data Type Conversion/1
  Override Switch3/1 -> Saturation 4-ent [0,1]/1
  override-4-ent/1 -> Override Switch3/1
  override-value-4-ent/1 -> Override Switch3/3
  override-4-bel/1 -> Override Switch2/1
  override-value-4-bel/1 -> Override Switch2/3
  u4-bel/1 -> Override Switch2/2
  Override Switch2/1 -> Saturation 4-bel [0,1]/1
  Saturation 4-bel [0,1]/1 -> Gain4/1  "Hub_Soll_B4P"
  Override Switch1/1 -> Saturation 2-ent [0,1]/1
  override-2-ent/1 -> Override Switch1/1
  override-value-2-ent/1 -> Override Switch1/3
  override-2-bel/1 -> Override Switch/1
  override-value-2-bel/1 -> Override Switch/3
  u2-bel/1 -> Override Switch/2
  Override Switch/1 -> Saturation 2-bel [0,1]/1
  Mux4/1 -> PositionBytes/1
  Saturation 2-bel [0,1]/1 -> Gain2/1  "Hub_Soll_B2P"
  u2-ent/1 -> Override Switch1/2
  u4-ent/1 -> Override Switch3/2
  Constant12/1 -> Multiport Switch/5
  Constant21/1 -> SteuerwortReglerByte1/1(Bit7)
  Constant20/1 -> SteuerwortReglerByte1/2(Bit6)
  Constant17/1 -> SteuerwortReglerByte1/3(Bit5)
  Constant30/1 -> SteuerwortReglerByte1/4(Bit4)
  Multiport Switch1/1 -> Demux5/1
  Demux5/2 -> SteuerwortReglerByte1/6(Bit2)
  Demux5/1 -> SteuerwortReglerByte1/5(Bit3)
  RegParB4/1 -> "1bis4 "/1
  Constant15/1 -> Multiport Switch1/4
  Constant16/1 -> Multiport Switch1/5
  Constant14/1 -> Multiport Switch1/3
  Constant18/1 -> Multiport Switch1/2
  "1bis4 "/1 -> Multiport Switch1/1
  RegParB2/1 -> 1bis4/1
  Demux4/2 -> SteuerwortReglerByte1/8(Bit0)
  Demux4/1 -> SteuerwortReglerByte1/7(Bit1)
  Multiport Switch/1 -> Demux4/1
  Constant11/1 -> Multiport Switch/4
  Constant10/1 -> Multiport Switch/3
  Constant9/1 -> Multiport Switch/2
  1bis4/1 -> Multiport Switch/1
  SteuerwortReglerByte1/1(U8Out) -> Data Type Conversion31/1
  Data Type Conversion31/1 -> Mux4/5

== system libbha_io/u2CAN ==
  u [-1,1] : Inport
  Override Switch : MultiPortSwitch  DataPortOrder=Zero-based contiguous  Inputs=2
  Saturation [-1,1] : Saturate  UpperLimit=1  LowerLimit=-1
  Saturation [0,1] : Saturate  UpperLimit=1  LowerLimit=0
  Sum2 : Sum  Inputs=|++  OutDataTypeStr=Inherit: Same as first input
  one : Constant
  override : Constant  Value=0
  override_value : Constant  Value=0.0
  to-0-1 : Gain  Gain=0.5  OutDataTypeStr=Inherit: Same as input  ParamDataTypeStr=Inherit: Same as input
  toCAN : Gain  Gain=8191  OutDataTypeStr=Inherit: Same as input  ParamDataTypeStr=Inherit: Same as input
  CAN : Outport
  wires:
  Saturation [0,1]/1 -> toCAN/1
  to-0-1/1 -> Saturation [0,1]/1
  Sum2/1 -> to-0-1/1
  one/1 -> Sum2/2
  toCAN/1 -> CAN/1
  Override Switch/1 -> Saturation [-1,1]/1
  u [-1,1]/1 -> Override Switch/2
  override_value/1 -> Override Switch/3
  override/1 -> Override Switch/1
  Saturation [-1,1]/1 -> Sum2/1

== system libbha_io/CalibrateLengthOffset/UseDefaultIfUseCalibration WithoutHavingCalibratedBefore ==
  state_calib : Inport
  LastValue : UnitDelay  SampleTime=-1
  MaxOfAll : MinMax  Function=max  Inputs=2
  Mux1 : Mux  Inputs=2
  Saturation : Saturate  UpperLimit=2  LowerLimit=0
  UseCalibration OnlyAllowed IfCalibratedOnce : Fcn  Expr=!(u(2)==0 ||(u(2)==1 && u(1)<2))*u(2)
  state_calib_allowed : Outport
  wires:
  state_calib/1 -> Saturation/1
  Saturation/1 -> MaxOfAll/2, Mux1/2
  LastValue/1 -> MaxOfAll/1
  Mux1/1 -> UseCalibration OnlyAllowed IfCalibratedOnce/1
  MaxOfAll/1 -> Mux1/1, LastValue/1
  UseCalibration OnlyAllowed IfCalibratedOnce/1 -> state_calib_allowed/1

== system libbha_io/CalibratePressureOffset/UseDefaultIfUseCalibration WithoutHavingCalibratedBefore ==
  state_calib : Inport
  LastValue : UnitDelay  SampleTime=-1
  MaxOfAll : MinMax  Function=max  Inputs=2
  Mux1 : Mux  Inputs=2
  Saturation : Saturate  UpperLimit=2  LowerLimit=0
  UseCalibration OnlyAllowed IfCalibratedOnce : Fcn  Expr=!(u(2)==0 ||(u(2)==1 && u(1)<2))*u(2)
  state_calib_allowed : Outport
  wires:
  state_calib/1 -> Saturation/1
  Saturation/1 -> MaxOfAll/2, Mux1/2
  LastValue/1 -> MaxOfAll/1
  Mux1/1 -> UseCalibration OnlyAllowed IfCalibratedOnce/1
  MaxOfAll/1 -> Mux1/1, LastValue/1
  UseCalibration OnlyAllowed IfCalibratedOnce/1 -> state_calib_allowed/1

== system libbha_io/Relative Skalierung/Triggered Subsystem ==
  In1 : Inport
  In2 : Inport  Port=2
  Trigger : TriggerPort
  Out1 : Outport  InitialOutput=x_min_init
  Out2 : Outport  Port=2  InitialOutput=x_min_init
  wires:
  In1/1 -> Out1/1
  In2/1 -> Out2/1

== system libbha_io/Relative Skalierung/Triggered Subsystem1 ==
  In1 : Inport
  In2 : Inport  Port=2
  Trigger : TriggerPort
  Out1 : Outport  InitialOutput=x_max_init
  Out2 : Outport  Port=2  InitialOutput=x_max_init
  wires:
  In1/1 -> Out1/1
  In2/1 -> Out2/1

== system libbha_io/Relative Skalierung (Ext)/Triggered Subsystem ==
  In1 : Inport
  In2 : Inport  Port=2
  Trigger : TriggerPort
  Out1 : Outport  InitialOutput=x_min_init
  Out2 : Outport  Port=2  InitialOutput=x_min_init
  wires:
  In2/1 -> Out2/1
  In1/1 -> Out1/1

== system libbha_io/Relative Skalierung (Ext)/Triggered Subsystem1 ==
  In1 : Inport
  In2 : Inport  Port=2
  Trigger : TriggerPort
  Out1 : Outport  InitialOutput=x_max_init
  Out2 : Outport  Port=2  InitialOutput=x_max_init
  wires:
  In2/1 -> Out2/1
  In1/1 -> Out1/1

== system libbha_io/Relative Skalierung (Ext)/calibrated_at_least_once ==
  calibration_active : Inport
  ena_min : Inport  Port=2
  ena_max : Inport  Port=3
  Logical Operator : Logic  Inputs=3  AllPortsSameDT=off  OutDataTypeStr=boolean
  not_calibrating : Logic  Operator=NOT  AllPortsSameDT=off  OutDataTypeStr=boolean
  was_enabled_once_max : Subsystem
  was_enabled_once_min : Subsystem
  calib_once_not_now : Outport
  wires:
  was_enabled_once_min/1(was_ena) -> Logical Operator/1
  ena_min/1 -> was_enabled_once_min/1(ena)
  was_enabled_once_max/1(was_ena) -> Logical Operator/2
  ena_max/1 -> was_enabled_once_max/1(ena)
  Logical Operator/1 -> calib_once_not_now/1
  calibration_active/1 -> not_calibrating/1
  not_calibrating/1 -> Logical Operator/3

== system libbha_io/u2Bytes-Valve-R2017.1/SteuerwortReglerByte1 ==
  Bit7 : Inport
  Bit6 : Inport  Port=2
  Bit5 : Inport  Port=3
  Bit4 : Inport  Port=4
  Bit3 : Inport  Port=5
  Bit2 : Inport  Port=6
  Bit1 : Inport  Port=7
  Bit0 : Inport  Port=8
  BitToU8 : Fcn  Expr=u(1)+2*u(2)+4*u(3)+8*u(4)+16*u(5)+32*u(6)+64*u(7)+128*u(8)
  Mux : Mux  Inputs=8
  U8Out : Outport
  wires:
  Bit5/1 -> Mux/6
  Bit4/1 -> Mux/5
  Bit0/1 -> Mux/1
  Bit2/1 -> Mux/3
  Bit1/1 -> Mux/2
  Bit3/1 -> Mux/4
  BitToU8/1 -> U8Out/1
  Bit7/1 -> Mux/8
  Bit6/1 -> Mux/7
  Mux/1 -> BitToU8/1

== system libbha_io/Relative Skalierung (Ext)/calibrated_at_least_once/was_enabled_once_max ==
  ena : Inport
  LastValue : UnitDelay  SampleTime=-1
  Logical Operator : Logic  Operator=OR  AllPortsSameDT=off  OutDataTypeStr=boolean
  was_ena : Outport
  wires:
  Logical Operator/1 -> LastValue/1, was_ena/1
  LastValue/1 -> Logical Operator/2
  ena/1 -> Logical Operator/1

== system libbha_io/Relative Skalierung (Ext)/calibrated_at_least_once/was_enabled_once_min ==
  ena : Inport
  LastValue : UnitDelay  SampleTime=-1
  Logical Operator : Logic  Operator=OR  AllPortsSameDT=off  OutDataTypeStr=boolean
  was_ena : Outport
  wires:
  ena/1 -> Logical Operator/1
  LastValue/1 -> Logical Operator/2
  Logical Operator/1 -> was_ena/1, LastValue/1

== matlab function libbha_io/overwrite split-u/select manual u ==
  data: u_pos input; u_neg input; u_set_pos output; u_man input; ena_u_man input; u_set_neg output
function [u_set_pos, u_set_neg] = select(u_pos, u_neg, u_man, ena_u_man)
%codegen

u_set_pos = u_pos;
u_set_neg = u_neg;
for i=1:length(ena_u_man)
   if ena_u_man(i) > 0.5
       u_set_pos(i) = max(0, u_man(i));
       u_set_neg(i) = max(0,-u_man(i));
   end
end

== matlab function libbha_io/Valves2SaveXDigital/is_positive ==
  data: in input; out output
function out = ispositive(in)
%#codegen

out = (in > 0);

== matlab function libbha_io/Relative Skalierung (Ext)/calc_gain_offset ==
  data: u1 input; gains output; u2 input; u3 input; u4 input; offsets output
function [gains,offsets] = calc_go(u1,u2,u3,u4)
%#codegen

gains   = (u4-u2)./(u3-u1);
offsets = (u3.*u2-u1.*u4)./(u3-u1);

== matlab function libbha_io/overwrite u/select manual u ==
  data: u input; u_set output; u_man input; ena_u_man input
function u_set = select(u, u_man, ena_u_man)
%codegen

u_set = u;
for i=1:length(u)
   if ena_u_man(i) > 0.5
       u_set(i) = u_man(i);
   end
end

== matlab function libbha_io/Relative Skalierung/calc_gain_offset ==
  data: u1 input; gains output; u2 input; u3 input; u4 input; offsets output
function [gains,offsets] = calc_go(u1,u2,u3,u4)
%#codegen

gains   = (u4-u2)./(u3-u1);
offsets = (u3.*u2-u1.*u4)./(u3-u1);
